simulink model "pole_fitted"  (R2021b)
settings: Solver=FixedStepAuto  StartTime=0.0  StopTime=5.0  FixedStep=0.01  RelTol=1e-3
libraries: fuzblock x1
settings Model: Creator=ПК  LastModifiedBy=ПК

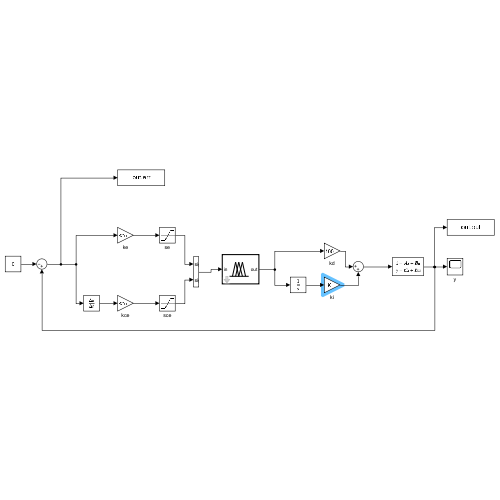
[thumbnail: Simulink's stored preview of the top-level diagram]
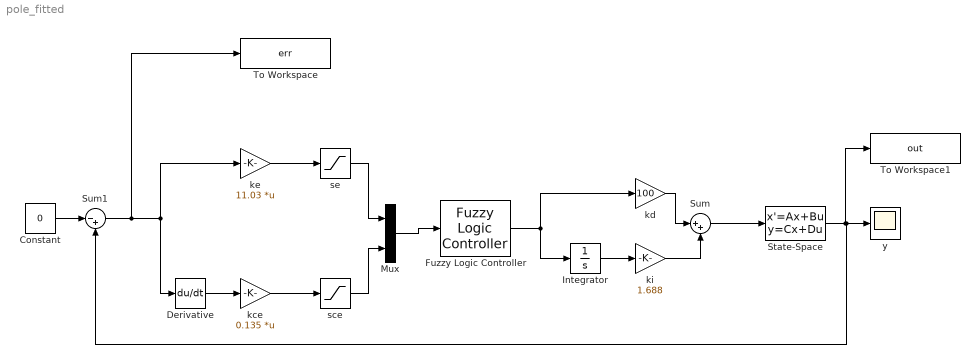
== system pole_fitted ==
  Constant : Constant  Value=0
  Derivative : Derivative
  Fuzzy Logic Controller : fuzblock/Fuzzy Logic  Controller  FIS='flc.fis'  OutputSampleNumber=101  DataType=double  FuzzifiedInputs=off  RuleFiringStrengths=off  RuleOutputs=off  AggregatedOutputs=off  SimulateUsing=Interpreted execution  OutOfRangeInputValueMessage=warning  NoRuleFiredMessage=warning  EmptyOutputFuzzySetMessage=warning
  Integrator : Integrator
  Mux : Mux  Inputs=2
      settings: DisplayOption=signals
  State-Space : StateSpace  A=[0 1 0 0; 0 0 -0.98 0; 0 0 0 1; 0 0 12.25 0]  B=[0; 0.5; 0; -6.25]  C=[0 0 1 0]  D=0  InitialCondition=[0 0 0.3 0]
  Sum : Sum  Inputs=|++
  Sum1 : Sum  Inputs=|-+
  To Workspace : ToWorkspace  VariableName=err  SampleTime=-1
  To Workspace1 : ToWorkspace  VariableName=out  SampleTime=-1
  kce : Gain  Gain=0.135  Multiplication=Matrix(K*u)
  kd : Gain  Gain=100
  ke : Gain  Gain=11.03  Multiplication=Matrix(K*u)
  ki : Gain  Gain=1.688
  sce : Saturate  UpperLimit=3  LowerLimit=-3
  se : Saturate  UpperLimit=3  LowerLimit=-3
  y : Scope
  wires:
  State-Space/1 -> To Workspace1/1, Sum1/2, y/1
  ke/1 -> se/1
  kce/1 -> sce/1
  se/1 -> Mux/1
  Mux/1 -> Fuzzy Logic Controller/1
  sce/1 -> Mux/2
  ki/1 -> Sum/2
  kd/1 -> Sum/1
  Sum/1 -> State-Space/1
  Integrator/1 -> ki/1
  Fuzzy Logic Controller/1 -> kd/1, Integrator/1
  Derivative/1 -> kce/1
  Constant/1 -> Sum1/1
  Sum1/1 -> To Workspace/1, ke/1, Derivative/1
